simulink model "EVTOLJOBYSIMULINKTHESISfinal"  (R2025a)
settings: Solver=VariableStepAuto  StartTime=0.0  StopTime=40  RelTol=1e-3
libraries: slpidlib x1, simulink x1
settings Model: Creator=Pc  LastModifiedBy=shubi

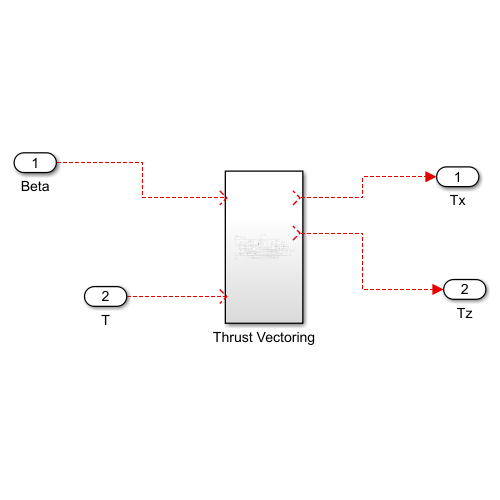
[thumbnail: Simulink's stored preview of the top-level diagram]
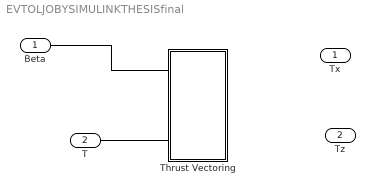
== system EVTOLJOBYSIMULINKTHESISfinal ==
  Beta : Inport
  T : Inport  Port=2
  Thrust Vectoring : Subsystem
  Tx : Outport
  Tz : Outport  Port=2
  wires:
  Beta/1 -> ?
  T/1 -> ?
  ? -> Tx/1
  ? -> Tz/1

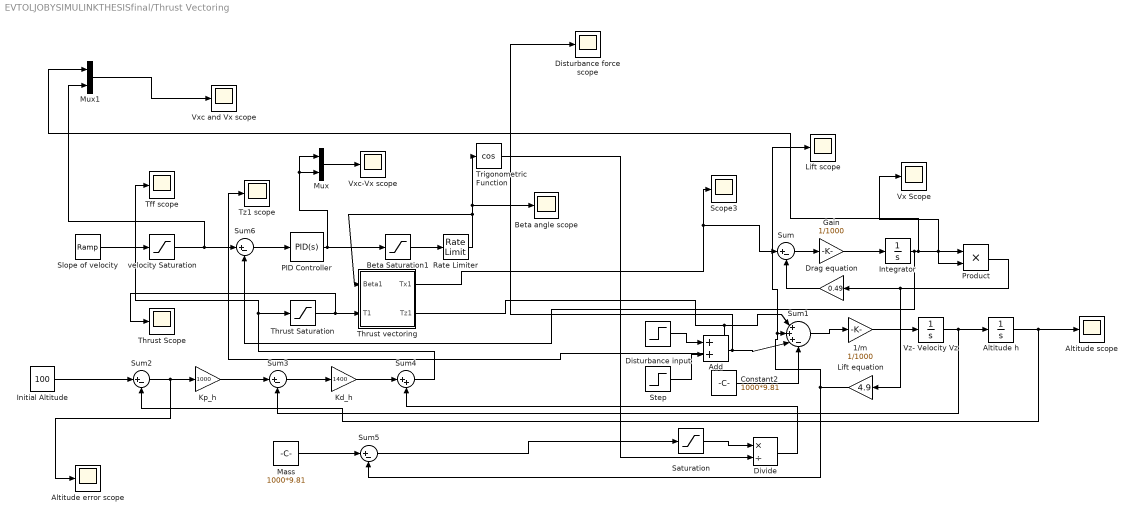
== system EVTOLJOBYSIMULINKTHESISfinal/Thrust Vectoring ==
  1/m : Gain  Gain=1/1000
  Add : Sum
  Altitude error scope : Scope
      settings: ActiveDisplayYMinimum=-1  ActiveDisplayYMaximum=1  DataLoggingVariableName=ScopeData8
  Altitude h : Integrator  InitialCondition=100
  Altitude scope : Scope
      settings: ActiveDisplayYMinimum=-1  ActiveDisplayYMaximum=1
  Beta Saturation1 : Saturate  UpperLimit=pi/3  LowerLimit=0
  Beta angle scope : Scope
      settings: ActiveDisplayYMinimum=-1  ActiveDisplayYMaximum=1  DataLoggingVariableName=ScopeData2
  Constant2 : Constant  Value=1000*9.81
  Disturbance force scope : Scope
      settings: ActiveDisplayYMinimum=-1  ActiveDisplayYMaximum=1  DataLoggingVariableName=ScopeData11
  Disturbance input : Step  Time=15  After=-500  SampleTime=0
  Divide : Product  Inputs=*/
  Drag equation : Gain  Gain=0.49
  Gain : Gain  Gain=1/1000
  Initial Altitude : Constant  Value=100
  Integrator : Integrator
  Kd_h : Gain  Gain=1400
  Kp_h : Gain  Gain=1000
  Lift equation : Gain  Gain=4.9
  Lift scope : Scope
      settings: ActiveDisplayYMinimum=-1247.4948680997413  ActiveDisplayYMaximum=9746.7601746264627  DataLoggingVariableName=ScopeData6
  Mass : Constant  Value=1000*9.81
  Mux : Mux  Inputs=2
  Mux1 : Mux  Inputs=2
  PID Controller : slpidlib/PID Controller  Controller=PID  Form=Parallel  TimeDomain=Continuous-time  UseExternalTs=off  SampleTime=-1  IntegratorMethod=Forward Euler  FilterMethod=Forward Euler  ControllerParametersSource=internal  P=0.02  I=0.005  UseKiTs=off  D=0  UseExternalDerivativeSource=off  N=100  UseFilter=on  TunerSelectOption=Transfer Function Based (PID Tuner App)  InitialConditionSource=internal  InitialConditionForIntegrator=0  InitialConditionForFilter=0  DifferentiatorICPrevScaledInput=0  ExternalReset=none  TrackingMode=off  Kt=1  LimitOutput=off  SatLimitsSource=internal  UpperSaturationLimit=inf  LowerSaturationLimit=-inf  LinearizeAsGain=on  AntiWindupMode=none  Kb=1  LimitIntegrator=off  UpperIntegratorSaturationLimit=inf  LowerIntegratorSaturationLimit=-inf  POutMin=[]  POutMax=[]  IOutMin=[]  IOutMax=[]  DOutMin=[]  DOutMax=[]  NOutMin=[]  NOutMax=[]  SumOutMin=[]  SumOutMax=[]  SaturationOutMin=[]  SaturationOutMax=[]  PParamMin=[]  PParamMax=[]  IParamMin=[]  IParamMax=[]  DParamMin=[]  DParamMax=[]  NParamMin=[]  NParamMax=[]  KbParamMin=[]  KbParamMax=[]  KtParamMin=[]  KtParamMax=[]  KbOutMin=[]  KbOutMax=[]  KtOutMin=[]  KtOutMax=[]  IntegratorOutMin=[]  IntegratorOutMax=[]  FilterOutMin=[]  FilterOutMax=[]  SumI1OutMin=[]  SumI1OutMax=[]  SumI2OutMin=[]  SumI2OutMax=[]  SumI3OutMin=[]  SumI3OutMax=[]  SumI4OutMin=[]  SumI4OutMax=[]  SumDOutMin=[]  SumDOutMax=[]  DifferentiatorOutMin=[]  DifferentiatorOutMax=[]  FilterDiffOutCoefMin=[]  FilterDiffOutCoefMax=[]  ReciprocalOutMin=[]  ReciprocalOutMax=[]  SumDenOutMin=[]  SumDenOutMax=[]  SumNumOutMin=[]  SumNumOutMax=[]  DivideOutMin=[]  DivideOutMax=[]  UdiffTsProdOutMin=[]  UdiffTsProdOutMax=[]  NTsProdOutMin=[]  NTsProdOutMax=[]  UintegralTsProdOutMin=[]  UintegralTsProdOutMax=[]  UngainTsProdOutMin=[]  UngainTsProdOutMax=[]  ClampingZeroOutDataTypeStr=Inherit: Inherit via back propagation  ClampingZeroOutMin=[]  ClampingZeroOutMax=[]  FilterDenConstantOutDataTypeStr=Inherit: Inherit via back propagation  FilterDenConstantOutMin=[]  FilterDenConstantOutMax=[]  PCopyOutDataTypeStr=Inherit: Inherit via back propagation  PCopyOutMin=[]  PCopyOutMax=[]  NCopyOutDataTypeStr=Inherit: Inherit via back propagation  NCopyOutMin=[]  NCopyOutMax=[]  IntegratorContinuousStateAttributes=''  IntegratorStateMustResolveToSignalObject=off  IntegratorRTWStateStorageClass=Auto  FilterContinuousStateAttributes=''  FilterStateMustResolveToSignalObject=off  FilterRTWStateStorageClass=Auto  ParallelPVariant=InternalParameters  IdealPVariant=Disabled  IVariant=InternalParameters  DVariant=InternalParameters  IntegratorVariant=Continuous  SatVariant=Disabled  AWVariant=Passthrough  PCopyVariant=Disabled  TRVariant=Disabled  FdbkBlocksVariant=Forward  IdealPFdbkVariant=Disabled  SatFdbkVariant=Disabled  DerivativeFilterVariant=ContFilter  NVariant=InternalParameters  NCopyVariant=Disabled  FilterICVariant=InternalICsFilter  IntegratorICVariant=InternalICs  ExternalResetVariant=Disabled  TRSumVariant=Passthrough  SumFdbkVariant=Disabled  SumVariant=Sum_PID  TsampFilterVariant=InternalTs  TsampNgainVariant=Passthrough  TsampIntegralVariant=Disabled_SignalSpec  ExternalSaturationOutDataTypeStr=Inherit: Same as second input  DerivativeSourceVariant=ErrorSignal  PreIntVariant=InternalPreInt
  Product : Product
  Rate Limiter : RateLimiter  RisingSlewLimit=5*pi/180  FallingSlewLimit=-5*pi/180  SampleTimeMode=inherited
  Saturation : Saturate  UpperLimit=inf  LowerLimit=0
  Scope3 : Scope
      settings: ActiveDisplayYMinimum=-1  ActiveDisplayYMaximum=1  DataLoggingVariableName=ScopeData3
  Slope of velocity : simulink/Sources/Ramp  slope=2  start=5  InitialOutput=0
  Step : Step  Time=20  After=500  SampleTime=0
  Sum{,2..3,5..6} (5 alike) : Sum  Inputs=|+-
  Sum1 : Sum  Inputs=|+++-
  Sum4 : Sum  Inputs=|++
  Tff scope : Scope
      settings: ActiveDisplayYMinimum=-1  ActiveDisplayYMaximum=1  DataLoggingVariableName=ScopeData7
  Thrust Saturation : Saturate  UpperLimit=20000  LowerLimit=0
  Thrust Scope : Scope
      settings: ActiveDisplayYMinimum=-1  ActiveDisplayYMaximum=1  DataLoggingVariableName=ScopeData5
  Thrust vectoring : Subsystem
  Trigonometric Function : Trigonometry  Operator=cos
  Tz1 scope : Scope
      settings: ActiveDisplayYMinimum=-0.13089969389957468  ActiveDisplayYMaximum=1.1780972450961724  DataLoggingVariableName=ScopeData4
  Vx Scope : Scope
      settings: ActiveDisplayYMinimum=-1  ActiveDisplayYMaximum=1
  Vxc and Vx scope : Scope
      settings: ActiveDisplayYMinimum=-1  ActiveDisplayYMaximum=1  DataLoggingVariableName=ScopeData10
  Vxc-Vx scope : Scope
      settings: ActiveDisplayYMinimum=-1  ActiveDisplayYMaximum=1  DataLoggingVariableName=ScopeData9
  Vz- Velocity Vz : Integrator
  velocity Saturation : Saturate  UpperLimit=40  LowerLimit=0
  wires:
  Sum/1 -> Gain/1
  Gain/1 -> Integrator/1
  Drag equation/1 -> Sum/2
  Integrator/1 -> Mux1/1, Product/2, Product/1, Vx Scope/1, Sum6/2
  Product/1 -> Lift equation/1, Drag equation/1
  Sum1/1 -> 1/m/1
  1/m/1 -> Vz- Velocity Vz/1
  Vz- Velocity Vz/1 -> Sum3/2, Altitude h/1
  Lift equation/1 -> Sum5/2, Lift scope/1, Sum1/2
  Altitude h/1 -> Sum2/2, Altitude scope/1
  Slope of velocity/1 -> velocity Saturation/1
  Thrust vectoring/2(Tz1) -> Tz1 scope/1, Sum1/1
  Thrust vectoring/1(Tx1) -> Sum/1, Scope3/1
  Initial Altitude/1 -> Sum2/1
  Sum2/1 -> Altitude error scope/1, Kp_h/1
  Kp_h/1 -> Sum3/1
  Sum3/1 -> Kd_h/1
  Kd_h/1 -> Sum4/1
  Sum4/1 -> Tff scope/1, Thrust Saturation/1
  Thrust Saturation/1 -> Thrust Scope/1, Thrust vectoring/2(T1)
  Mass/1 -> Sum5/1
  Trigonometric Function/1 -> Divide/2
  Divide/1 -> Sum4/2
  Sum5/1 -> Saturation/1
  Saturation/1 -> Divide/1
  velocity Saturation/1 -> Mux1/2, Sum6/1
  Sum6/1 -> PID Controller/1
  PID Controller/1 -> Mux/1, Mux/2, Beta Saturation1/1
  Beta Saturation1/1 -> Rate Limiter/1
  Rate Limiter/1 -> Thrust vectoring/1(Beta1), Trigonometric Function/1, Beta angle scope/1
  Mux/1 -> Vxc-Vx scope/1
  Mux1/1 -> Vxc and Vx scope/1
  Constant2/1 -> Sum1/4
  Disturbance input/1 -> Add/1
  Step/1 -> Add/2
  Add/1 -> Disturbance force scope/1, Sum1/3

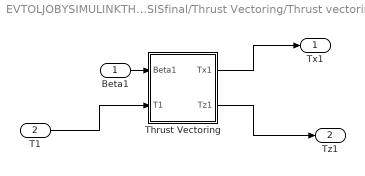
== system EVTOLJOBYSIMULINKTHESISfinal/Thrust Vectoring/Thrust vectoring ==
  Beta1 : Inport
  T1 : Inport  Port=2
  Thrust Vectoring : Subsystem
  Tx1 : Outport
  Tz1 : Outport  Port=2
  wires:
  T1/1 -> Thrust Vectoring/2(T1)
  Thrust Vectoring/2(Tz1) -> Tz1/1
  Thrust Vectoring/1(Tx1) -> Tx1/1
  Beta1/1 -> Thrust Vectoring/1(Beta1)

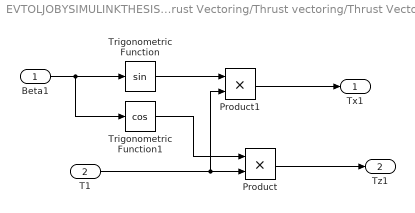
== system EVTOLJOBYSIMULINKTHESISfinal/Thrust Vectoring/Thrust vectoring/Thrust Vectoring ==
  Beta1 : Inport
  T1 : Inport  Port=2
  Product : Product
  Product1 : Product
  Trigonometric Function : Trigonometry
  Trigonometric Function1 : Trigonometry  Operator=cos
  Tx1 : Outport
  Tz1 : Outport  Port=2
  wires:
  Beta1/1 -> Trigonometric Function/1, Trigonometric Function1/1
  Trigonometric Function/1 -> Product1/1
  T1/1 -> Product1/2, Product/2
  Product/1 -> Tz1/1
  Trigonometric Function1/1 -> Product/1
  Product1/1 -> Tx1/1
